simulink model "Asservissement_modele_non_simplifie"  (R2019b)
settings: Solver=VariableStepAuto  StartTime=0.0  StopTime=10.0  RelTol=1e-3
undefined symbols (not defined in the file): Cr, f, J, Ke, Km, R
libraries: simulink x1
settings Model: Creator=Shanly  LastModifiedBy=Shanly

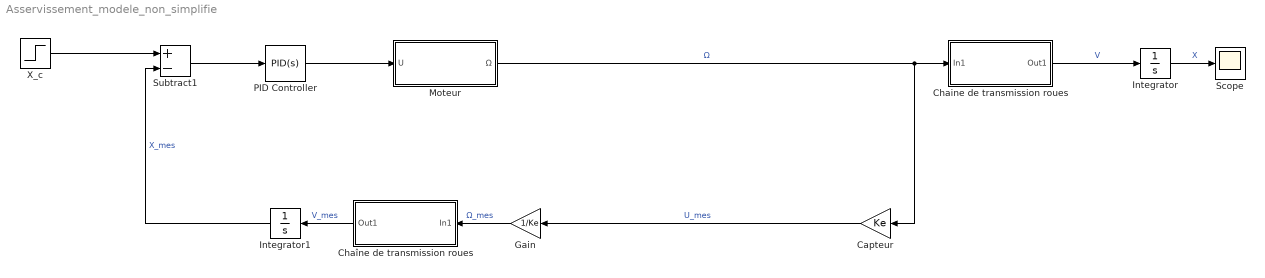
== system Asservissement_modele_non_simplifie ==
  "Capteur " : Gain  Gain=Ke
  Chaine de transmission roues : Subsystem
  Chaîne de transmission roues : Subsystem
  Gain : Gain  Gain=1/Ke
  Integrator : Integrator
  Integrator1 : Integrator
  "Moteur " : Subsystem
  PID Controller : simulink/Continuous/PID Controller  Controller=PID  Form=Parallel  TimeDomain=Continuous-time  SampleTime=-1  IntegratorMethod=Forward Euler  FilterMethod=Forward Euler  ControllerParametersSource=internal  P=0.31  I=0.395  D=-0.02  UseFilter=on  N=4.13  TunerSelectOption=Transfer Function Based (PID Tuner App)  InitialConditionSource=internal  InitialConditionForIntegrator=0  InitialConditionForFilter=0  DifferentiatorICPrevScaledInput=0  ExternalReset=none  TrackingMode=off  Kt=1  LimitOutput=off  UpperSaturationLimit=inf  LowerSaturationLimit=-inf  LinearizeAsGain=on  AntiWindupMode=none  Kb=1  POutMin=[]  POutMax=[]  IOutMin=[]  IOutMax=[]  DOutMin=[]  DOutMax=[]  NOutMin=[]  NOutMax=[]  SumOutMin=[]  SumOutMax=[]  SaturationOutMin=[]  SaturationOutMax=[]  PParamMin=[]  PParamMax=[]  IParamMin=[]  IParamMax=[]  DParamMin=[]  DParamMax=[]  NParamMin=[]  NParamMax=[]  KbParamMin=[]  KbParamMax=[]  KtParamMin=[]  KtParamMax=[]  KbOutMin=[]  KbOutMax=[]  KtOutMin=[]  KtOutMax=[]  IntegratorOutMin=[]  IntegratorOutMax=[]  FilterOutMin=[]  FilterOutMax=[]  SumI1OutMin=[]  SumI1OutMax=[]  SumI2OutMin=[]  SumI2OutMax=[]  SumI3OutMin=[]  SumI3OutMax=[]  SumI4OutMin=[]  SumI4OutMax=[]  SumDOutMin=[]  SumDOutMax=[]  DifferentiatorOutMin=[]  DifferentiatorOutMax=[]  FilterDiffOutCoefMin=[]  FilterDiffOutCoefMax=[]  ReciprocalOutMin=[]  ReciprocalOutMax=[]  SumDenOutMin=[]  SumDenOutMax=[]  SumNumOutMin=[]  SumNumOutMax=[]  DivideOutMin=[]  DivideOutMax=[]  IntegratorContinuousStateAttributes=''  IntegratorStateMustResolveToSignalObject=off  IntegratorRTWStateStorageClass=Auto  FilterContinuousStateAttributes=''  FilterStateMustResolveToSignalObject=off  FilterRTWStateStorageClass=Auto  ParallelPVariant=InternalParameters  IdealPVariant=Disabled  IVariant=InternalParameters  DVariant=InternalParameters  IntegratorVariant=Continuous  SatVariant=Disabled  AWVariant=Passthrough  PCopyVariant=Disabled  TRVariant=Disabled  FdbkBlocksVariant=Forward  IdealPFdbkVariant=Disabled  SatFdbkVariant=Disabled  DerivativeFilterVariant=ContFilter  NVariant=InternalParameters  NCopyVariant=Disabled  FilterICVariant=InternalICsFilter  IntegratorICVariant=InternalICs  ExternalResetVariant=Disabled  TRSumVariant=Passthrough  SumFdbkVariant=Disabled  SumVariant=Sum_PID
  Scope : Scope
  Subtract1 : Sum  Inputs=+-
  X_c : Step  SampleTime=0
  wires:
  "Moteur "/1(Ω) -> "Capteur "/1, Chaine de transmission roues/1(In1)  "Ω"
  PID Controller/1 -> "Moteur "/1(U)
  Chaine de transmission roues/1(Out1) -> Integrator/1  "V"
  Integrator/1 -> Scope/1  "X"
  X_c/1 -> Subtract1/1
  "Capteur "/1 -> Gain/1  "U_mes"
  Gain/1 -> Chaîne de transmission roues/1(In1)  "Ω_mes"
  Chaîne de transmission roues/1(Out1) -> Integrator1/1  "V_mes"
  Integrator1/1 -> Subtract1/2  "X_mes"
  Subtract1/1 -> PID Controller/1

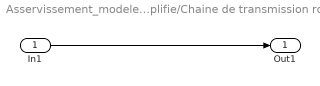
== system Asservissement_modele_non_simplifie/Chaine de transmission roues ==
  In1 : Inport
  Out1 : Outport
  wires:
  In1/1 -> Out1/1

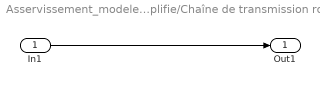
== system Asservissement_modele_non_simplifie/Chaîne de transmission roues ==
  In1 : Inport
  Out1 : Outport
  wires:
  In1/1 -> Out1/1

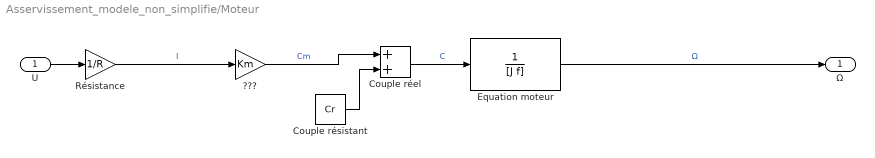
== system Asservissement_modele_non_simplifie/Moteur  ==
  U : Inport
  "???" : Gain  Gain=Km
  Couple réel : Sum
  Couple résistant : Constant  Value=Cr
  Equation moteur : TransferFcn  Denominator=[J f]
  Résistance : Gain  Gain=1/R
  Ω : Outport
  wires:
  U/1 -> Résistance/1
  Equation moteur/1 -> Ω/1  "Ω"
  Résistance/1 -> "???"/1  "I"
  "???"/1 -> Couple réel/1  "Cm"
  Couple réel/1 -> Equation moteur/1  "C"
  Couple résistant/1 -> Couple réel/2
